simulink model "einfacher_Prozess"  (Simulink 7.5)
settings: Solver=ode45  StartTime=0.0  StopTime=10.0  RelTol=1e-3
settings Model: Creator=Mattse  LastModifiedBy=Mattse
settings DebuggingCC: FcnCallInpInsideContextMsg=Enable All

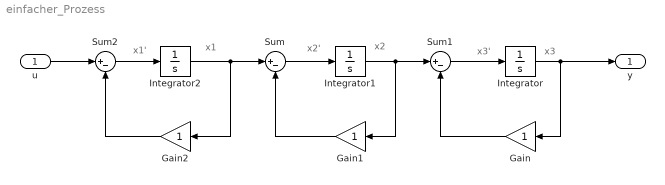
== system einfacher_Prozess ==
  note: x1'
  note: x1
  note: x2'
  note: x2
  note: x3'
  note: x3
  u : Inport
  Gain : Gain
  Gain1 : Gain
  Gain2 : Gain
  Integrator : Integrator
  Integrator1 : Integrator
  Integrator2 : Integrator
  Sum : Sum  Inputs=|+-
  Sum1 : Sum  Inputs=|+-
  Sum2 : Sum  Inputs=|+-
  y : Outport
  wires:
  Integrator1/1 -> Sum1/1, Gain1/1
  Sum1/1 -> Integrator/1
  Sum/1 -> Integrator1/1
  Integrator2/1 -> Sum/1, Gain2/1
  Sum2/1 -> Integrator2/1
  u/1 -> Sum2/1
  Integrator/1 -> Gain/1, y/1
  Gain/1 -> Sum1/2
  Gain1/1 -> Sum/2
  Gain2/1 -> Sum2/2
